simulink model "BU01AM"  (R2018b)
settings: Solver=FixedStepAuto  StartTime=0.0  StopTime=10.0  FixedStep=0.02  RelTol=1e-3
model workspace (MAT data in the model file):
  B = 1.94
  C = 1.94
  Clp = -0.3
  Clr = 0
  Cly = 0
  Cmq1 = -1.95
  Cmq2 = 1.56
  Cmx1 = -0.631
  Cmx2 = 0
  Cmz1 = -0.29
  Cmz2 = 0.18
  Cnp = 0
  Cnr = -0.19
  Cx1 = -0.142
  Cy = -0.384
  Cyp = 0
  Cyr = 0
  Cz1 = -1.91
  Cz2 = 1.69
  Czq1 = 0
  Czq2 = 0
  Czx1 = -0.771
  Czx2 = 0
  S = 0.4
libraries: simulink x3
settings Model: Creator=39926  LastModifiedBy=39926

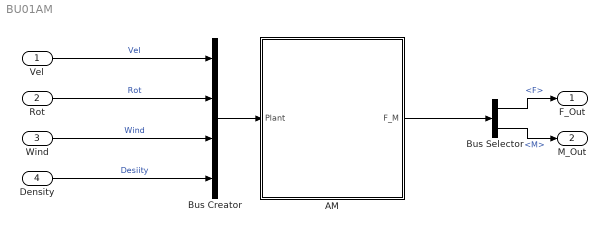
== system BU01AM ==
  Vel : Inport  PortDimensions=3
  Rot : Inport  Port=2  PortDimensions=3
  Wind : Inport  Port=3  PortDimensions=3
  Density : Inport  Port=4  PortDimensions=1
  AM : Subsystem  mask{Cx1=-0.142, Cx2=0.140, Cy=-0.384, Cyp=0.0, Cyr=0.0, Cz1=-1.91, Cz2=1.69, Czx1=-0.771, Czx2=0.0, Czq1=0.0, Czq2=0.0, Clp=-0.3, Cly=0.0, Clr=0.0, Cmq1=-1.95, Cmq2=1.56, Cmz1=-0.29, Cmz2=0.18, Cmx1=-0.631, Cmx2=0.0, Cnp=0.0, Cnr=-0.19, Cny=0.0151, S=0.4, B=1.94, C=0.21}
      mask prompts: Cx1 "前飞X轴向力系数Cx1"; Cx2 "后飞X轴向力系数Cx2"; Cy "侧向力系数Cy"; Cyp "滚转引起侧向力系数Cyp"; Cyr "偏航引起侧向力系数Cyr"; Cz1 "下降Z轴向力系数Cz1"; Cz2 "爬升Z轴向力系数Cz2"; Czx1 "前飞Z轴向力系数Czx1"; Czx2 "后飞Z轴向力系数Czx2"; Czq1 "抬头Z轴向力系数Czq1"; Czq2 "低头Z轴向力系数Czq2"; Clp "滚转阻尼Clp"; Cly "横向运动引起的滚转力矩系数Cly"; Clr "偏航运动引起的滚转力矩系数Clr"; Cmq1 "抬头运动俯仰阻尼Cmq1"; Cmq2 "低头运动俯仰阻尼Cmq2"; Cmz1 "垂直下降时俯仰力矩系数Cmz1"; Cmz2 "垂直爬升时俯仰力矩系数Cmz2"; Cmx1 "前飞时俯仰力矩系数Cmx1"; Cmx2 "后飞时俯仰力矩系数Cmx2"; Cnp "滚转引起的偏航力矩系数Cnp"; Cnr "偏航阻尼"; Cny "横向运动引起的偏航力矩系数Cny"; S "机翼面积S"; B "翼展B"; C "弦长C"
      mask Display: disp('机体气动模型');
  Bus Selector : BusSelector  OutputSignals=F,M
  Bus Creator : BusCreator  Inputs=4
  F_Out : Outport
  M_Out : Outport  Port=2
  wires:
  Vel/1 -> Bus Creator/1  "Vel"
  Rot/1 -> Bus Creator/2  "Rot"
  Wind/1 -> Bus Creator/3  "Wind"
  Density/1 -> Bus Creator/4  "Desiity"
  Bus Creator/1 -> AM/1(Plant)
  AM/1(F_M) -> Bus Selector/1
  Bus Selector/1 -> F_Out/1  "<F>"
  Bus Selector/2 -> M_Out/1  "<M>"

== system BU01AM/AM ==
  Plant : Inport
  Bus Selector : BusSelector  OutputSignals=Vel,Wind,Desiity,Rot
  Sum : Sum  Inputs=|+-
  求解气动力 : Subsystem
  F_M : Outport
  wires:
  Plant/1 -> Bus Selector/1
  Bus Selector/1 -> Sum/1  "<Vel>"
  Bus Selector/2 -> Sum/2  "<Wind>"
  Sum/1 -> 求解气动力/1(Vel_real)
  Bus Selector/3 -> 求解气动力/2(Density)  "<Desiity>"
  Bus Selector/4 -> 求解气动力/3(Rot)  "<Rot>"
  求解气动力/1(F_M) -> F_M/1

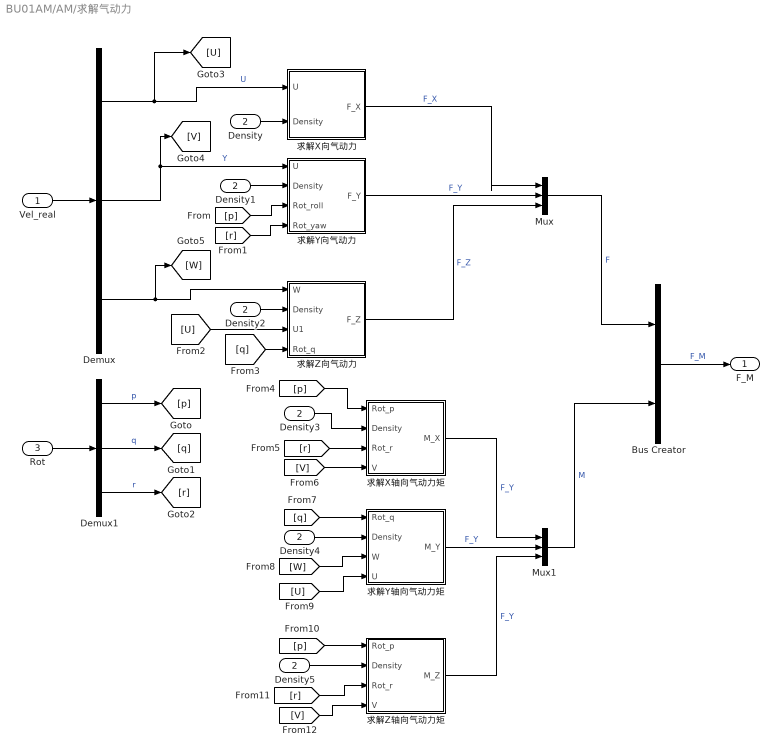
== system BU01AM/AM/求解气动力 ==
  Vel_real : Inport
  Density : Inport  Port=2
  Rot : Inport  Port=3
  Bus Creator : BusCreator  Inputs=2
  Demux : Demux  Outputs=3
  Demux1 : Demux  Outputs=3
  Density{1..5} (5 alike) : InportShadow  Port=2
  Mux : Mux  Inputs=3
  Mux1 : Mux  Inputs=3
  求解X向气动力 : Subsystem
  求解X轴向气动力矩 : Subsystem
  求解Y向气动力 : Subsystem
  求解Y轴向气动力矩 : Subsystem
  求解Z向气动力 : Subsystem
  求解Z轴向气动力矩 : Subsystem
  F_M : Outport
  wires:
  Vel_real/1 -> Demux/1
  Demux/1 -> [U], 求解X向气动力/1(U)  "U"
  Density/1 -> 求解X向气动力/2(Density)
  Demux/2 -> [V], 求解Y向气动力/1(U)  "Y"
  Density1/1 -> 求解Y向气动力/2(Density)
  Rot/1 -> Demux1/1
  Demux1/1 -> [p]  "p"
  Demux1/2 -> [q]  "q"
  Demux1/3 -> [r]  "r"
  [p] -> 求解Y向气动力/3(Rot_roll)
  [r] -> 求解Y向气动力/4(Rot_yaw)
  Demux/3 -> [W], 求解Z向气动力/1(W)
  [U] -> 求解Z向气动力/3(U1)
  Density2/1 -> 求解Z向气动力/2(Density)
  [q] -> 求解Z向气动力/4(Rot_q)
  求解X向气动力/1(F_X) -> Mux/1  "F_X"
  求解Y向气动力/1(F_Y) -> Mux/2  "F_Y"
  求解Z向气动力/1("F_Z ") -> Mux/3  "F_Z"
  [p] -> 求解X轴向气动力矩/1(Rot_p)
  Density3/1 -> 求解X轴向气动力矩/2(Density)
  [r] -> 求解X轴向气动力矩/3(Rot_r)
  [V] -> 求解X轴向气动力矩/4(V)
  [q] -> 求解Y轴向气动力矩/1(Rot_q)
  Density4/1 -> 求解Y轴向气动力矩/2(Density)
  [W] -> 求解Y轴向气动力矩/3(W)
  [U] -> 求解Y轴向气动力矩/4(U)
  [p] -> 求解Z轴向气动力矩/1(Rot_p)
  Density5/1 -> 求解Z轴向气动力矩/2(Density)
  [r] -> 求解Z轴向气动力矩/3(Rot_r)
  [V] -> 求解Z轴向气动力矩/4(V)
  求解X轴向气动力矩/1(M_X) -> Mux1/1  "F_Y"
  求解Y轴向气动力矩/1(M_Y) -> Mux1/2  "F_Y"
  求解Z轴向气动力矩/1(M_Z) -> Mux1/3  "F_Y"
  Mux/1 -> Bus Creator/1  "F"
  Mux1/1 -> Bus Creator/2  "M"
  Bus Creator/1 -> F_M/1  "F_M"

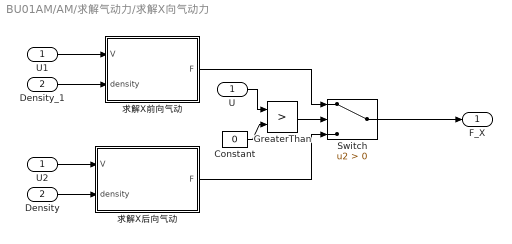
== system BU01AM/AM/求解气动力/求解X向气动力 ==
  U : Inport
  Density : Inport  Port=2
  Constant : Constant  Value=0
  Density_1 : InportShadow  Port=2
  GreaterThan : RelationalOperator  Operator=>  OutDataTypeStr=boolean  RndMeth=Simplest
  Switch : Switch  Criteria=u2 > Threshold
  U1 : InportShadow
  U2 : InportShadow
  求解X前向气动 : Subsystem  mask{S=S, C=Cx1}
      mask Display: disp('计算空气力矩')
  求解X后向气动 : Subsystem  mask{S=S, C=Cx2}
      mask Display: disp('计算空气力矩')
  F_X : Outport
  wires:
  Density/1 -> 求解X后向气动/2(density)
  求解X前向气动/1(F) -> Switch/1
  Density_1/1 -> 求解X前向气动/2(density)
  U/1 -> GreaterThan/1
  Constant/1 -> GreaterThan/2
  U1/1 -> 求解X前向气动/1(V)
  U2/1 -> 求解X后向气动/1(V)
  GreaterThan/1 -> Switch/2
  求解X后向气动/1(F) -> Switch/3
  Switch/1 -> F_X/1

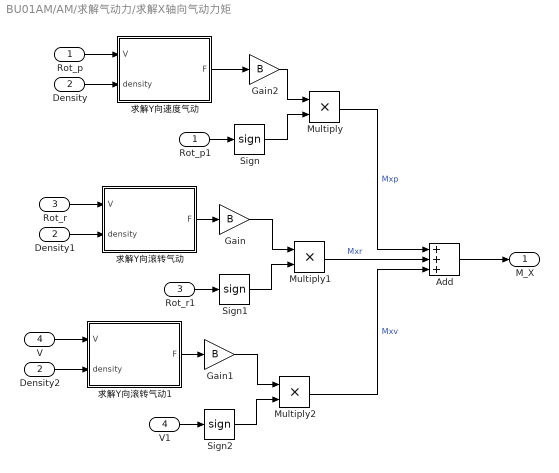
== system BU01AM/AM/求解气动力/求解X轴向气动力矩 ==
  Rot_p : Inport
  Density : Inport  Port=2
  Rot_r : Inport  Port=3
  V : Inport  Port=4
  Add : Sum  Inputs=3
  Density1 : InportShadow  Port=2
  Density2 : InportShadow  Port=2
  Gain : Gain  Gain=B
  Gain1 : Gain  Gain=B
  Gain2 : Gain  Gain=B
  Multiply : Product
  Multiply1 : Product
  Multiply2 : Product
  Rot_p1 : InportShadow
  "Rot_r1 " : InportShadow  Port=3
  Sign : Signum
  Sign1 : Signum
  Sign2 : Signum
  V1 : InportShadow  Port=4
  求解Y向滚转气动 : Subsystem  mask{S=S, C=Clr}
      mask Display: disp('计算空气力矩')
  求解Y向滚转气动1 : Subsystem  mask{S=S, C=Cly}
      mask Display: disp('计算空气力矩')
  求解Y向速度气动 : Subsystem  mask{S=S, C=Clp}
      mask Display: disp('计算空气力矩')
  M_X : Outport
  wires:
  Add/1 -> M_X/1
  Multiply2/1 -> Add/3  "Mxv"
  Multiply1/1 -> Add/2  "Mxr"
  Sign2/1 -> Multiply2/2
  V1/1 -> Sign2/1
  Density2/1 -> 求解Y向滚转气动1/2(density)
  V/1 -> 求解Y向滚转气动1/1(V)
  求解Y向滚转气动1/1(F) -> Gain1/1
  Gain1/1 -> Multiply2/1
  Gain/1 -> Multiply1/1
  求解Y向滚转气动/1(F) -> Gain/1
  Multiply/1 -> Add/1  "Mxp"
  Rot_r/1 -> 求解Y向滚转气动/1(V)
  Density1/1 -> 求解Y向滚转气动/2(density)
  "Rot_r1 "/1 -> Sign1/1
  Sign1/1 -> Multiply1/2
  Sign/1 -> Multiply/2
  Rot_p1/1 -> Sign/1
  Density/1 -> 求解Y向速度气动/2(density)
  Rot_p/1 -> 求解Y向速度气动/1(V)
  求解Y向速度气动/1(F) -> Gain2/1
  Gain2/1 -> Multiply/1

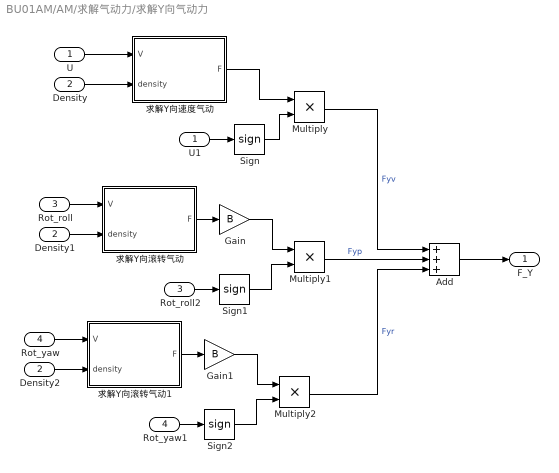
== system BU01AM/AM/求解气动力/求解Y向气动力 ==
  U : Inport
  Density : Inport  Port=2
  Rot_roll : Inport  Port=3
  Rot_yaw : Inport  Port=4
  Add : Sum  Inputs=3
  Density1 : InportShadow  Port=2
  Density2 : InportShadow  Port=2
  Gain : Gain  Gain=B
  Gain1 : Gain  Gain=B
  Multiply : Product
  Multiply1 : Product
  Multiply2 : Product
  Rot_roll2 : InportShadow  Port=3
  Rot_yaw1 : InportShadow  Port=4
  Sign : Signum
  Sign1 : Signum
  Sign2 : Signum
  U1 : InportShadow
  求解Y向滚转气动 : Subsystem  mask{S=S, C=Cyp}
      mask Display: disp('计算空气力矩')
  求解Y向滚转气动1 : Subsystem  mask{S=S, C=Cyr}
      mask Display: disp('计算空气力矩')
  求解Y向速度气动 : Subsystem  mask{S=S, C=Cy}
      mask Display: disp('计算空气力矩')
  F_Y : Outport
  wires:
  U/1 -> 求解Y向速度气动/1(V)
  Density/1 -> 求解Y向速度气动/2(density)
  求解Y向速度气动/1(F) -> Multiply/1
  U1/1 -> Sign/1
  Sign/1 -> Multiply/2
  Sign1/1 -> Multiply1/2
  Rot_roll2/1 -> Sign1/1
  Density1/1 -> 求解Y向滚转气动/2(density)
  Rot_roll/1 -> 求解Y向滚转气动/1(V)
  Multiply/1 -> Add/1  "Fyv"
  求解Y向滚转气动/1(F) -> Gain/1
  Gain/1 -> Multiply1/1
  Gain1/1 -> Multiply2/1
  求解Y向滚转气动1/1(F) -> Gain1/1
  Rot_yaw/1 -> 求解Y向滚转气动1/1(V)
  Density2/1 -> 求解Y向滚转气动1/2(density)
  Rot_yaw1/1 -> Sign2/1
  Sign2/1 -> Multiply2/2
  Multiply1/1 -> Add/2  "Fyp"
  Multiply2/1 -> Add/3  "Fyr"
  Add/1 -> F_Y/1

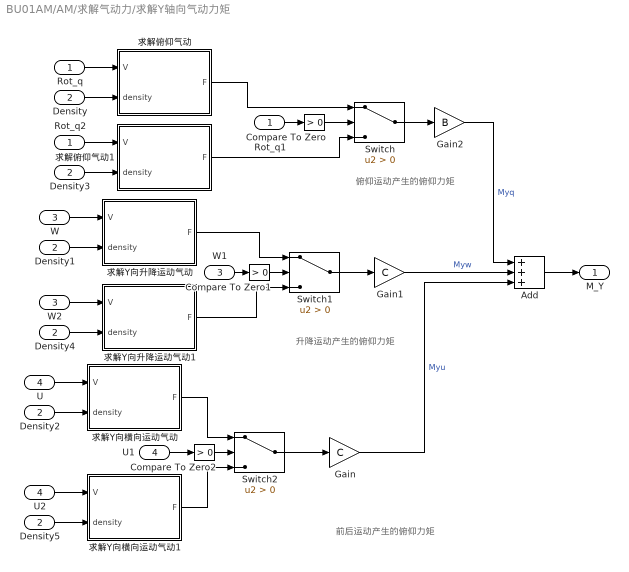
== system BU01AM/AM/求解气动力/求解Y轴向气动力矩 ==
  note: 前后运动产生的俯仰力矩
  note: 升降运动产生的俯仰力矩
  note: 俯仰运动产生的俯仰力矩
  Rot_q : Inport
  Density : Inport  Port=2
  W : Inport  Port=3
  U : Inport  Port=4
  Add : Sum  Inputs=3
  Compare To Zero : simulink/Logic and Bit Operations/Compare To Zero  relop=>  OutDataTypeStr=boolean
  Compare To Zero1 : simulink/Logic and Bit Operations/Compare To Zero  relop=>  OutDataTypeStr=boolean
  Compare To Zero2 : simulink/Logic and Bit Operations/Compare To Zero  relop=>  OutDataTypeStr=boolean
  Density{1..5} (5 alike) : InportShadow  Port=2
  Gain : Gain  Gain=C
  Gain1 : Gain  Gain=C
  Gain2 : Gain  Gain=B
  Rot_q1 : InportShadow
  Rot_q2 : InportShadow
  Switch : Switch  Criteria=u2 > Threshold
  Switch1 : Switch  Criteria=u2 > Threshold
  Switch2 : Switch  Criteria=u2 > Threshold
  U1 : InportShadow  Port=4
  U2 : InportShadow  Port=4
  W1 : InportShadow  Port=3
  W2 : InportShadow  Port=3
  求解Y向升降运动气动 : Subsystem  mask{S=S, C=Cmz1}
      mask Display: disp('计算空气力矩')
  求解Y向升降运动气动1 : Subsystem  mask{S=S, C=Cmz2}
      mask Display: disp('计算空气力矩')
  求解Y向横向运动气动 : Subsystem  mask{S=S, C=Cmx1}
      mask Display: disp('计算空气力矩')
  求解Y向横向运动气动1 : Subsystem  mask{S=S, C=Cmx2}
      mask Display: disp('计算空气力矩')
  求解俯仰气动 : Subsystem  mask{S=S, C=Cmq1}
      mask Display: disp('计算空气力矩')
  求解俯仰气动1 : Subsystem  mask{S=S, C=Cmq2}
      mask Display: disp('计算空气力矩')
  M_Y : Outport
  wires:
  求解俯仰气动/1(F) -> Switch/1
  Rot_q/1 -> 求解俯仰气动/1(V)
  Density/1 -> 求解俯仰气动/2(density)
  Density1/1 -> 求解Y向升降运动气动/2(density)
  W/1 -> 求解Y向升降运动气动/1(V)
  求解Y向横向运动气动/1(F) -> Switch2/1
  U/1 -> 求解Y向横向运动气动/1(V)
  Density2/1 -> 求解Y向横向运动气动/2(density)
  Add/1 -> M_Y/1
  求解俯仰气动1/1(F) -> Switch/3
  Rot_q1/1 -> Compare To Zero/1
  Compare To Zero/1 -> Switch/2
  Rot_q2/1 -> 求解俯仰气动1/1(V)
  Density3/1 -> 求解俯仰气动1/2(density)
  求解Y向升降运动气动/1(F) -> Switch1/1
  W1/1 -> Compare To Zero1/1
  Compare To Zero1/1 -> Switch1/2
  求解Y向升降运动气动1/1(F) -> Switch1/3
  W2/1 -> 求解Y向升降运动气动1/1(V)
  Density4/1 -> 求解Y向升降运动气动1/2(density)
  U1/1 -> Compare To Zero2/1
  Compare To Zero2/1 -> Switch2/2
  求解Y向横向运动气动1/1(F) -> Switch2/3
  U2/1 -> 求解Y向横向运动气动1/1(V)
  Density5/1 -> 求解Y向横向运动气动1/2(density)
  Switch2/1 -> Gain/1
  Switch1/1 -> Gain1/1
  Gain1/1 -> Add/2  "Myw"
  Gain/1 -> Add/3  "Myu"
  Switch/1 -> Gain2/1
  Gain2/1 -> Add/1  "Myq"

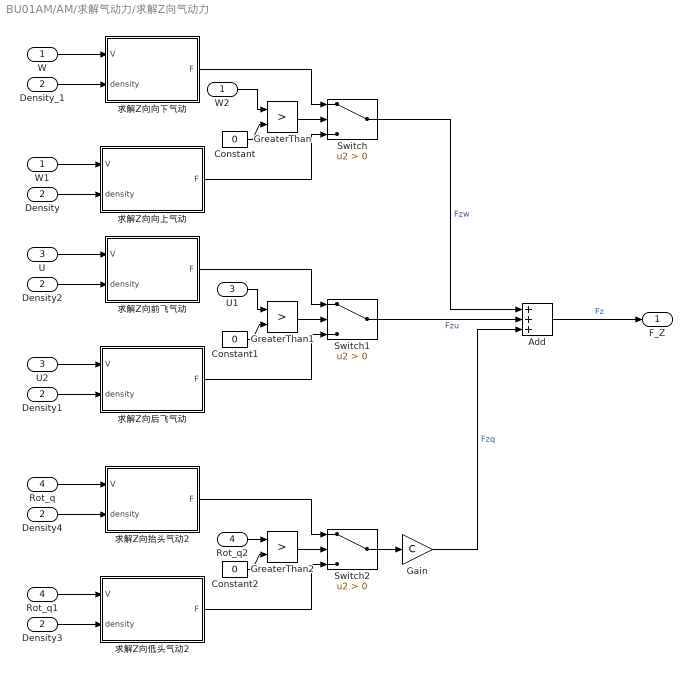
== system BU01AM/AM/求解气动力/求解Z向气动力 ==
  W : Inport
  Density : Inport  Port=2
  U1 : Inport  Port=3
  Rot_q : Inport  Port=4
  Add : Sum  Inputs=3
  Constant : Constant  Value=0
  Constant1 : Constant  Value=0
  Constant2 : Constant  Value=0
  Density{1..4} (4 alike) : InportShadow  Port=2
  Density_1 : InportShadow  Port=2
  Gain : Gain  Gain=C
  GreaterThan : RelationalOperator  Operator=>  OutDataTypeStr=boolean  RndMeth=Simplest
  GreaterThan1 : RelationalOperator  Operator=>  OutDataTypeStr=boolean  RndMeth=Simplest
  GreaterThan2 : RelationalOperator  Operator=>  OutDataTypeStr=boolean  RndMeth=Simplest
  Rot_q1 : InportShadow  Port=4
  Rot_q2 : InportShadow  Port=4
  Switch : Switch  Criteria=u2 > Threshold
  Switch1 : Switch  Criteria=u2 > Threshold
  Switch2 : Switch  Criteria=u2 > Threshold
  U : InportShadow  Port=3
  U2 : InportShadow  Port=3
  W1 : InportShadow
  W2 : InportShadow
  求解Z向低头气动2 : Subsystem  mask{S=S, C=Czq2}
      mask Display: disp('计算空气力矩')
  求解Z向前飞气动 : Subsystem  mask{S=S, C=Czx1}
      mask Display: disp('计算空气力矩')
  求解Z向后飞气动 : Subsystem  mask{S=S, C=Czx2}
      mask Display: disp('计算空气力矩')
  求解Z向向上气动 : Subsystem  mask{S=S, C=Cz2}
      mask Display: disp('计算空气力矩')
  求解Z向向下气动 : Subsystem  mask{S=S, C=Cz1}
      mask Display: disp('计算空气力矩')
  求解Z向抬头气动2 : Subsystem  mask{S=S, C=Czq1}
      mask Display: disp('计算空气力矩')
  "F_Z " : Outport
  wires:
  Switch/1 -> Add/1  "Fzw"
  求解Z向向上气动/1(F) -> Switch/3
  GreaterThan/1 -> Switch/2
  W1/1 -> 求解Z向向上气动/1(V)
  W/1 -> 求解Z向向下气动/1(V)
  Constant/1 -> GreaterThan/2
  W2/1 -> GreaterThan/1
  Density_1/1 -> 求解Z向向下气动/2(density)
  求解Z向向下气动/1(F) -> Switch/1
  Density/1 -> 求解Z向向上气动/2(density)
  Density1/1 -> 求解Z向后飞气动/2(density)
  求解Z向前飞气动/1(F) -> Switch1/1
  Density2/1 -> 求解Z向前飞气动/2(density)
  U1/1 -> GreaterThan1/1
  Constant1/1 -> GreaterThan1/2
  U/1 -> 求解Z向前飞气动/1(V)
  U2/1 -> 求解Z向后飞气动/1(V)
  GreaterThan1/1 -> Switch1/2
  求解Z向后飞气动/1(F) -> Switch1/3
  Switch1/1 -> Add/2  "Fzu"
  求解Z向低头气动2/1(F) -> Switch2/3
  GreaterThan2/1 -> Switch2/2
  Rot_q1/1 -> 求解Z向低头气动2/1(V)
  Rot_q/1 -> 求解Z向抬头气动2/1(V)
  Constant2/1 -> GreaterThan2/2
  Rot_q2/1 -> GreaterThan2/1
  Density4/1 -> 求解Z向抬头气动2/2(density)
  求解Z向抬头气动2/1(F) -> Switch2/1
  Density3/1 -> 求解Z向低头气动2/2(density)
  Switch2/1 -> Gain/1
  Gain/1 -> Add/3  "Fzq"
  Add/1 -> "F_Z "/1  "Fz"

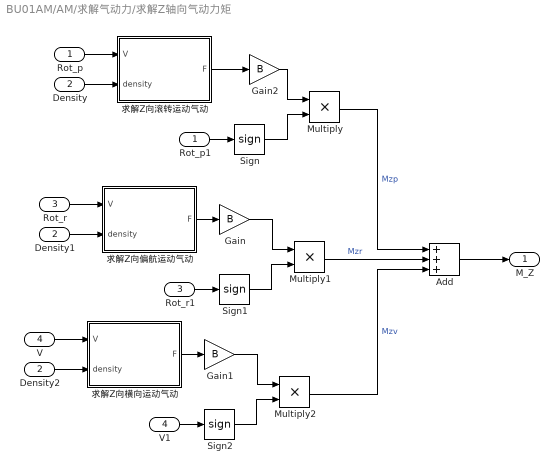
== system BU01AM/AM/求解气动力/求解Z轴向气动力矩 ==
  Rot_p : Inport
  Density : Inport  Port=2
  Rot_r : Inport  Port=3
  V : Inport  Port=4
  Add : Sum  Inputs=3
  Density1 : InportShadow  Port=2
  Density2 : InportShadow  Port=2
  Gain : Gain  Gain=B
  Gain1 : Gain  Gain=B
  Gain2 : Gain  Gain=B
  Multiply : Product
  Multiply1 : Product
  Multiply2 : Product
  Rot_p1 : InportShadow
  "Rot_r1 " : InportShadow  Port=3
  Sign : Signum
  Sign1 : Signum
  Sign2 : Signum
  V1 : InportShadow  Port=4
  求解Z向偏航运动气动 : Subsystem  mask{S=S, C=Cnr}
      mask Display: disp('计算空气力矩')
  求解Z向横向运动气动 : Subsystem  mask{S=S, C=0.0151}
      mask Display: disp('计算空气力矩')
  求解Z向滚转运动气动 : Subsystem  mask{S=S, C=Cnp}
      mask Display: disp('计算空气力矩')
  M_Z : Outport
  wires:
  Gain2/1 -> Multiply/1
  求解Z向滚转运动气动/1(F) -> Gain2/1
  Rot_p/1 -> 求解Z向滚转运动气动/1(V)
  Density/1 -> 求解Z向滚转运动气动/2(density)
  Rot_p1/1 -> Sign/1
  Sign/1 -> Multiply/2
  Sign1/1 -> Multiply1/2
  "Rot_r1 "/1 -> Sign1/1
  Density1/1 -> 求解Z向偏航运动气动/2(density)
  Rot_r/1 -> 求解Z向偏航运动气动/1(V)
  Multiply/1 -> Add/1  "Mzp"
  求解Z向偏航运动气动/1(F) -> Gain/1
  Gain/1 -> Multiply1/1
  Gain1/1 -> Multiply2/1
  求解Z向横向运动气动/1(F) -> Gain1/1
  V/1 -> 求解Z向横向运动气动/1(V)
  Density2/1 -> 求解Z向横向运动气动/2(density)
  V1/1 -> Sign2/1
  Sign2/1 -> Multiply2/2
  Multiply1/1 -> Add/2  "Mzr"
  Multiply2/1 -> Add/3  "Mzv"
  Add/1 -> M_Z/1

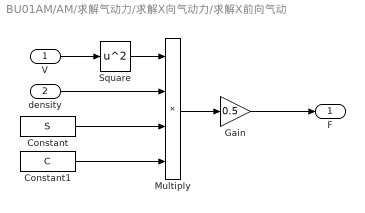
== system BU01AM/AM/求解气动力/求解X向气动力/求解X前向气动 ==
  V : Inport
  density : Inport  Port=2
  Constant : Constant  Value=S
  Constant1 : Constant  Value=C
  Gain : Gain  Gain=0.5
  Multiply : Product  Inputs=4
  Square : Math  Operator=square  SaturateOnIntegerOverflow=on
  F : Outport
  wires:
  V/1 -> Square/1
  Square/1 -> Multiply/1
  density/1 -> Multiply/2
  Constant/1 -> Multiply/3
  Constant1/1 -> Multiply/4
  Multiply/1 -> Gain/1
  Gain/1 -> F/1

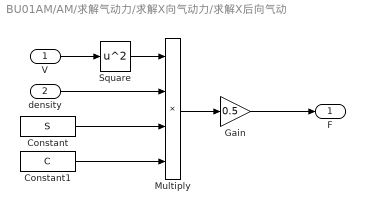
== system BU01AM/AM/求解气动力/求解X向气动力/求解X后向气动 ==
  V : Inport
  density : Inport  Port=2
  Constant : Constant  Value=S
  Constant1 : Constant  Value=C
  Gain : Gain  Gain=0.5
  Multiply : Product  Inputs=4
  Square : Math  Operator=square  SaturateOnIntegerOverflow=on
  F : Outport
  wires:
  Gain/1 -> F/1
  Multiply/1 -> Gain/1
  Constant1/1 -> Multiply/4
  Constant/1 -> Multiply/3
  density/1 -> Multiply/2
  Square/1 -> Multiply/1
  V/1 -> Square/1

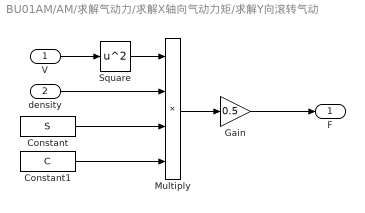
== system BU01AM/AM/求解气动力/求解X轴向气动力矩/求解Y向滚转气动 ==
  V : Inport
  density : Inport  Port=2
  Constant : Constant  Value=S
  Constant1 : Constant  Value=C
  Gain : Gain  Gain=0.5
  Multiply : Product  Inputs=4
  Square : Math  Operator=square  SaturateOnIntegerOverflow=on
  F : Outport
  wires:
  Gain/1 -> F/1
  Multiply/1 -> Gain/1
  Constant1/1 -> Multiply/4
  Constant/1 -> Multiply/3
  density/1 -> Multiply/2
  Square/1 -> Multiply/1
  V/1 -> Square/1

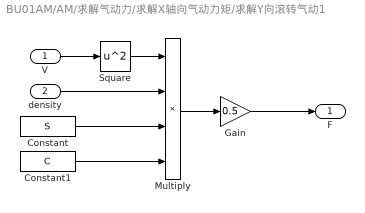
== system BU01AM/AM/求解气动力/求解X轴向气动力矩/求解Y向滚转气动1 ==
  V : Inport
  density : Inport  Port=2
  Constant : Constant  Value=S
  Constant1 : Constant  Value=C
  Gain : Gain  Gain=0.5
  Multiply : Product  Inputs=4
  Square : Math  Operator=square  SaturateOnIntegerOverflow=on
  F : Outport
  wires:
  V/1 -> Square/1
  Square/1 -> Multiply/1
  density/1 -> Multiply/2
  Constant/1 -> Multiply/3
  Constant1/1 -> Multiply/4
  Multiply/1 -> Gain/1
  Gain/1 -> F/1

== system BU01AM/AM/求解气动力/求解X轴向气动力矩/求解Y向速度气动 ==
  V : Inport
  density : Inport  Port=2
  Constant : Constant  Value=S
  Constant1 : Constant  Value=C
  Gain : Gain  Gain=0.5
  Multiply : Product  Inputs=4
  Square : Math  Operator=square  SaturateOnIntegerOverflow=on
  F : Outport
  wires:
  V/1 -> Square/1
  Square/1 -> Multiply/1
  density/1 -> Multiply/2
  Constant/1 -> Multiply/3
  Constant1/1 -> Multiply/4
  Multiply/1 -> Gain/1
  Gain/1 -> F/1

== system BU01AM/AM/求解气动力/求解Y向气动力/求解Y向滚转气动 ==
  V : Inport
  density : Inport  Port=2
  Constant : Constant  Value=S
  Constant1 : Constant  Value=C
  Gain : Gain  Gain=0.5
  Multiply : Product  Inputs=4
  Square : Math  Operator=square  SaturateOnIntegerOverflow=on
  F : Outport
  wires:
  V/1 -> Square/1
  Square/1 -> Multiply/1
  density/1 -> Multiply/2
  Constant/1 -> Multiply/3
  Constant1/1 -> Multiply/4
  Multiply/1 -> Gain/1
  Gain/1 -> F/1

== system BU01AM/AM/求解气动力/求解Y向气动力/求解Y向滚转气动1 ==
  V : Inport
  density : Inport  Port=2
  Constant : Constant  Value=S
  Constant1 : Constant  Value=C
  Gain : Gain  Gain=0.5
  Multiply : Product  Inputs=4
  Square : Math  Operator=square  SaturateOnIntegerOverflow=on
  F : Outport
  wires:
  Gain/1 -> F/1
  Multiply/1 -> Gain/1
  Constant1/1 -> Multiply/4
  Constant/1 -> Multiply/3
  density/1 -> Multiply/2
  Square/1 -> Multiply/1
  V/1 -> Square/1

== system BU01AM/AM/求解气动力/求解Y向气动力/求解Y向速度气动 ==
  V : Inport
  density : Inport  Port=2
  Constant : Constant  Value=S
  Constant1 : Constant  Value=C
  Gain : Gain  Gain=0.5
  Multiply : Product  Inputs=4
  Square : Math  Operator=square  SaturateOnIntegerOverflow=on
  F : Outport
  wires:
  Gain/1 -> F/1
  Multiply/1 -> Gain/1
  Constant1/1 -> Multiply/4
  Constant/1 -> Multiply/3
  density/1 -> Multiply/2
  Square/1 -> Multiply/1
  V/1 -> Square/1

== system BU01AM/AM/求解气动力/求解Y轴向气动力矩/求解Y向升降运动气动 ==
  V : Inport
  density : Inport  Port=2
  Constant : Constant  Value=S
  Constant1 : Constant  Value=C
  Gain : Gain  Gain=0.5
  Multiply : Product  Inputs=4
  Square : Math  Operator=square  SaturateOnIntegerOverflow=on
  F : Outport
  wires:
  V/1 -> Square/1
  Square/1 -> Multiply/1
  density/1 -> Multiply/2
  Constant/1 -> Multiply/3
  Constant1/1 -> Multiply/4
  Multiply/1 -> Gain/1
  Gain/1 -> F/1

== system BU01AM/AM/求解气动力/求解Y轴向气动力矩/求解Y向升降运动气动1 ==
  V : Inport
  density : Inport  Port=2
  Constant : Constant  Value=S
  Constant1 : Constant  Value=C
  Gain : Gain  Gain=0.5
  Multiply : Product  Inputs=4
  Square : Math  Operator=square  SaturateOnIntegerOverflow=on
  F : Outport
  wires:
  Gain/1 -> F/1
  Multiply/1 -> Gain/1
  Constant1/1 -> Multiply/4
  Constant/1 -> Multiply/3
  density/1 -> Multiply/2
  Square/1 -> Multiply/1
  V/1 -> Square/1

== system BU01AM/AM/求解气动力/求解Y轴向气动力矩/求解Y向横向运动气动 ==
  V : Inport
  density : Inport  Port=2
  Constant : Constant  Value=S
  Constant1 : Constant  Value=C
  Gain : Gain  Gain=0.5
  Multiply : Product  Inputs=4
  Square : Math  Operator=square  SaturateOnIntegerOverflow=on
  F : Outport
  wires:
  Gain/1 -> F/1
  Multiply/1 -> Gain/1
  Constant1/1 -> Multiply/4
  Constant/1 -> Multiply/3
  density/1 -> Multiply/2
  Square/1 -> Multiply/1
  V/1 -> Square/1

== system BU01AM/AM/求解气动力/求解Y轴向气动力矩/求解Y向横向运动气动1 ==
  V : Inport
  density : Inport  Port=2
  Constant : Constant  Value=S
  Constant1 : Constant  Value=C
  Gain : Gain  Gain=0.5
  Multiply : Product  Inputs=4
  Square : Math  Operator=square  SaturateOnIntegerOverflow=on
  F : Outport
  wires:
  V/1 -> Square/1
  Square/1 -> Multiply/1
  density/1 -> Multiply/2
  Constant/1 -> Multiply/3
  Constant1/1 -> Multiply/4
  Multiply/1 -> Gain/1
  Gain/1 -> F/1

== system BU01AM/AM/求解气动力/求解Y轴向气动力矩/求解俯仰气动 ==
  V : Inport
  density : Inport  Port=2
  Constant : Constant  Value=S
  Constant1 : Constant  Value=C
  Gain : Gain  Gain=0.5
  Multiply : Product  Inputs=4
  Square : Math  Operator=square  SaturateOnIntegerOverflow=on
  F : Outport
  wires:
  Gain/1 -> F/1
  Multiply/1 -> Gain/1
  Constant1/1 -> Multiply/4
  Constant/1 -> Multiply/3
  density/1 -> Multiply/2
  Square/1 -> Multiply/1
  V/1 -> Square/1

== system BU01AM/AM/求解气动力/求解Y轴向气动力矩/求解俯仰气动1 ==
  V : Inport
  density : Inport  Port=2
  Constant : Constant  Value=S
  Constant1 : Constant  Value=C
  Gain : Gain  Gain=0.5
  Multiply : Product  Inputs=4
  Square : Math  Operator=square  SaturateOnIntegerOverflow=on
  F : Outport
  wires:
  V/1 -> Square/1
  Square/1 -> Multiply/1
  density/1 -> Multiply/2
  Constant/1 -> Multiply/3
  Constant1/1 -> Multiply/4
  Multiply/1 -> Gain/1
  Gain/1 -> F/1

== system BU01AM/AM/求解气动力/求解Z向气动力/求解Z向低头气动2 ==
  V : Inport
  density : Inport  Port=2
  Constant : Constant  Value=S
  Constant1 : Constant  Value=C
  Gain : Gain  Gain=0.5
  Multiply : Product  Inputs=4
  Square : Math  Operator=square  SaturateOnIntegerOverflow=on
  F : Outport
  wires:
  V/1 -> Square/1
  Square/1 -> Multiply/1
  density/1 -> Multiply/2
  Constant/1 -> Multiply/3
  Constant1/1 -> Multiply/4
  Multiply/1 -> Gain/1
  Gain/1 -> F/1

== system BU01AM/AM/求解气动力/求解Z向气动力/求解Z向前飞气动 ==
  V : Inport
  density : Inport  Port=2
  Constant : Constant  Value=S
  Constant1 : Constant  Value=C
  Gain : Gain  Gain=0.5
  Multiply : Product  Inputs=4
  Square : Math  Operator=square  SaturateOnIntegerOverflow=on
  F : Outport
  wires:
  V/1 -> Square/1
  Square/1 -> Multiply/1
  density/1 -> Multiply/2
  Constant/1 -> Multiply/3
  Constant1/1 -> Multiply/4
  Multiply/1 -> Gain/1
  Gain/1 -> F/1

== system BU01AM/AM/求解气动力/求解Z向气动力/求解Z向后飞气动 ==
  V : Inport
  density : Inport  Port=2
  Constant : Constant  Value=S
  Constant1 : Constant  Value=C
  Gain : Gain  Gain=0.5
  Multiply : Product  Inputs=4
  Square : Math  Operator=square  SaturateOnIntegerOverflow=on
  F : Outport
  wires:
  Gain/1 -> F/1
  Multiply/1 -> Gain/1
  Constant1/1 -> Multiply/4
  Constant/1 -> Multiply/3
  density/1 -> Multiply/2
  Square/1 -> Multiply/1
  V/1 -> Square/1

== system BU01AM/AM/求解气动力/求解Z向气动力/求解Z向向上气动 ==
  V : Inport
  density : Inport  Port=2
  Constant : Constant  Value=S
  Constant1 : Constant  Value=C
  Gain : Gain  Gain=0.5
  Multiply : Product  Inputs=4
  Square : Math  Operator=square  SaturateOnIntegerOverflow=on
  F : Outport
  wires:
  V/1 -> Square/1
  Square/1 -> Multiply/1
  density/1 -> Multiply/2
  Constant/1 -> Multiply/3
  Constant1/1 -> Multiply/4
  Multiply/1 -> Gain/1
  Gain/1 -> F/1

== system BU01AM/AM/求解气动力/求解Z向气动力/求解Z向向下气动 ==
  V : Inport
  density : Inport  Port=2
  Constant : Constant  Value=S
  Constant1 : Constant  Value=C
  Gain : Gain  Gain=0.5
  Multiply : Product  Inputs=4
  Square : Math  Operator=square  SaturateOnIntegerOverflow=on
  F : Outport
  wires:
  Gain/1 -> F/1
  Multiply/1 -> Gain/1
  Constant1/1 -> Multiply/4
  Constant/1 -> Multiply/3
  density/1 -> Multiply/2
  Square/1 -> Multiply/1
  V/1 -> Square/1

== system BU01AM/AM/求解气动力/求解Z向气动力/求解Z向抬头气动2 ==
  V : Inport
  density : Inport  Port=2
  Constant : Constant  Value=S
  Constant1 : Constant  Value=C
  Gain : Gain  Gain=0.5
  Multiply : Product  Inputs=4
  Square : Math  Operator=square  SaturateOnIntegerOverflow=on
  F : Outport
  wires:
  Gain/1 -> F/1
  Multiply/1 -> Gain/1
  Constant1/1 -> Multiply/4
  Constant/1 -> Multiply/3
  density/1 -> Multiply/2
  Square/1 -> Multiply/1
  V/1 -> Square/1

== system BU01AM/AM/求解气动力/求解Z轴向气动力矩/求解Z向偏航运动气动 ==
  V : Inport
  density : Inport  Port=2
  Constant : Constant  Value=S
  Constant1 : Constant  Value=C
  Gain : Gain  Gain=0.5
  Multiply : Product  Inputs=4
  Square : Math  Operator=square  SaturateOnIntegerOverflow=on
  F : Outport
  wires:
  V/1 -> Square/1
  Square/1 -> Multiply/1
  density/1 -> Multiply/2
  Constant/1 -> Multiply/3
  Constant1/1 -> Multiply/4
  Multiply/1 -> Gain/1
  Gain/1 -> F/1

== system BU01AM/AM/求解气动力/求解Z轴向气动力矩/求解Z向横向运动气动 ==
  V : Inport
  density : Inport  Port=2
  Constant : Constant  Value=S
  Constant1 : Constant  Value=C
  Gain : Gain  Gain=0.5
  Multiply : Product  Inputs=4
  Square : Math  Operator=square  SaturateOnIntegerOverflow=on
  F : Outport
  wires:
  Gain/1 -> F/1
  Multiply/1 -> Gain/1
  Constant1/1 -> Multiply/4
  Constant/1 -> Multiply/3
  density/1 -> Multiply/2
  Square/1 -> Multiply/1
  V/1 -> Square/1

== system BU01AM/AM/求解气动力/求解Z轴向气动力矩/求解Z向滚转运动气动 ==
  V : Inport
  density : Inport  Port=2
  Constant : Constant  Value=S
  Constant1 : Constant  Value=C
  Gain : Gain  Gain=0.5
  Multiply : Product  Inputs=4
  Square : Math  Operator=square  SaturateOnIntegerOverflow=on
  F : Outport
  wires:
  Gain/1 -> F/1
  Multiply/1 -> Gain/1
  Constant1/1 -> Multiply/4
  Constant/1 -> Multiply/3
  density/1 -> Multiply/2
  Square/1 -> Multiply/1
  V/1 -> Square/1
